simulink model "dcmtrCtrl_PID_Harness2"  (R2022b)
settings: Solver=FixedStepAuto  StartTime=0.0  StopTime=10  FixedStep=Ctrl_Ts  RelTol=1e-3
libraries: simulink_extras x2
settings Model: DataDictionary=dcmtr_ctrl.sldd  Creator=smuckati  LastModifiedBy=smuckati
settings OptimizationCC: DefaultParameterBehavior=Inlined  UseDivisionForNetSlopeComputation=on  EnhancedBackFolding=on  PassReuseOutputArgsAs=Individual arguments  ZeroExternalMemoryAtStartup=off  ZeroInternalMemoryAtStartup=off  OptimizeBlockOrder=speed  DifferentSizesBufferReuse=on  OptimizationCustomize=off  EfficientTunableParamExpr=on
settings DebuggingCC: SignalRangeChecking=error  ParameterPrecisionLossMsg=none  ParameterTunabilityLossMsg=error  UnconnectedInputMsg=warning  UnconnectedOutputMsg=warning  UnconnectedLineMsg=warning
settings ModelReferenceCC: EnableRefExpFcnMdlSchedulingChecks=on
settings SFSimCC: MATLABDynamicMemAlloc=off
settings RTWCC: Description=Embedded Coder  SystemTargetFile=ert.tlc  GenCodeOnly=on  TemplateMakefile=ert_default_tmf  CodeExecutionProfiling=on  CodeProfilingSaveOptions=AllData  CodeProfilingInstrumentation=detailed  DLArmComputeVersion=19.05
settings CodeAppCC: ForceParamTrailComments=on  IgnoreCustomStorageClasses=off  OperatorAnnotations=on  SimulinkDataObjDesc=on  SFDataObjDesc=on  InsertBlockDesc=on
settings ERTTargetCC: TargetLangStandard=C99 (ISO)  GenerateSampleERTMain=on  InlinedParameterPlacement=NonHierarchical  ERTCustomFileTemplate=example_file_process.tlc

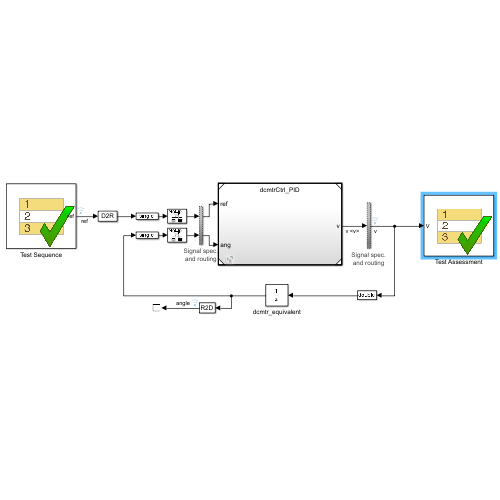
[thumbnail: Simulink's stored preview of the top-level diagram]
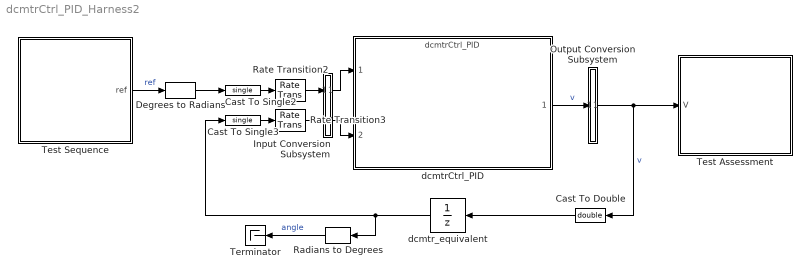
== system dcmtrCtrl_PID_Harness2 ==
  Cast To Double : DataTypeConversion  OutDataTypeStr=double  SaturateOnIntegerOverflow=off  RndMeth=Floor
  Cast To Single2 : DataTypeConversion  OutDataTypeStr=single  SaturateOnIntegerOverflow=off  RndMeth=Floor
  Cast To Single3 : DataTypeConversion  OutDataTypeStr=single  SaturateOnIntegerOverflow=off  RndMeth=Floor
  Degrees to Radians : simulink_extras/Transformations/Degrees to Radians
  Input Conversion Subsystem : Subsystem  Tag=__SLT_ICS__  Description=|
      | Signal spec.
      | and routing
      settings: AttributesFormatString=%<Description>
  Output Conversion Subsystem : Subsystem  Tag=__SLT_OCS__  Description=|
      | Signal spec.
      | and routing
      settings: AttributesFormatString=%<Description>
  Radians to Degrees : simulink_extras/Transformations/Radians to Degrees
  Rate Transition2 : RateTransition  OutPortSampleTime=Ctrl_Ts
  Rate Transition3 : RateTransition  OutPortSampleTime=Ctrl_Ts
  Terminator : Terminator
  Test Assessment : Test Sequence  TreatAsAtomicUnit=on
  Test Sequence : Test Sequence  TreatAsAtomicUnit=on
  dcmtrCtrl_PID : ModelReference  ModelNameDialog=dcmtrCtrl_PID  SimulationMode=Normal  ModelReferenceVersion=3.0
  dcmtr_equivalent : UnitDelay  SampleTime=-1  HasFrameUpgradeWarning=on
  wires:
  Degrees to Radians/1 -> Cast To Single2/1
  Output Conversion Subsystem/1(Outport_1) -> Cast To Double/1, Test Assessment/1(V)  "v"
  Input Conversion Subsystem/1(Outport_1) -> dcmtrCtrl_PID/1
  Input Conversion Subsystem/2(Outport_2) -> dcmtrCtrl_PID/2
  dcmtrCtrl_PID/1 -> Output Conversion Subsystem/1(Inport_1)  "v"
  Cast To Single2/1 -> Rate Transition2/1
  Rate Transition2/1 -> Input Conversion Subsystem/1(Inport_1)
  Cast To Single3/1 -> Rate Transition3/1
  Rate Transition3/1 -> Input Conversion Subsystem/2(Inport_2)
  dcmtr_equivalent/1 -> Radians to Degrees/1, Cast To Single3/1
  Cast To Double/1 -> dcmtr_equivalent/1
  Test Sequence/1(ref) -> Degrees to Radians/1  "ref"
  Radians to Degrees/1 -> Terminator/1  "angle"

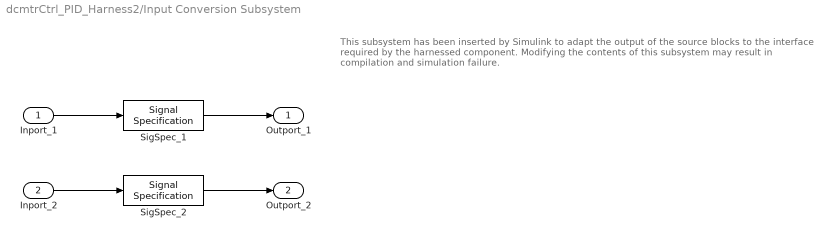
== system dcmtrCtrl_PID_Harness2/Input Conversion Subsystem ==
  note: This subsystem has been inserted by Simulink to adapt the output of the source blocks to the interface required by the harnessed component.
      |  Modifying the contents of this subsystem may result in compilation and simulation failure.
  Inport_1 : Inport
  Inport_2 : Inport  Port=2
  SigSpec_1 : SignalSpecification  OutDataTypeStr=single  Dimensions=[1]  SampleTime=0.01
  SigSpec_2 : SignalSpecification  OutDataTypeStr=single  Dimensions=[1]  SampleTime=0.01
  Outport_1 : Outport
  Outport_2 : Outport  Port=2
  wires:
  SigSpec_1/1 -> Outport_1/1
  Inport_1/1 -> SigSpec_1/1
  SigSpec_2/1 -> Outport_2/1
  Inport_2/1 -> SigSpec_2/1

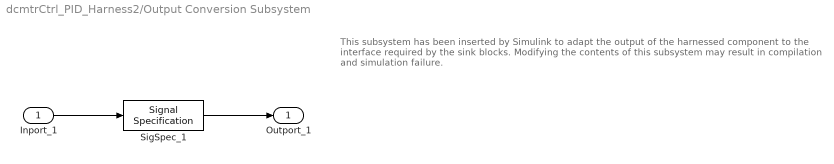
== system dcmtrCtrl_PID_Harness2/Output Conversion Subsystem ==
  note: This subsystem has been inserted by Simulink to adapt the output of the harnessed component to the interface required by the sink blocks.
      |  Modifying the contents of this subsystem may result in compilation and simulation failure.
  Inport_1 : Inport
  SigSpec_1 : SignalSpecification  OutDataTypeStr=single  Dimensions=[1]  SampleTime=0.01
  Outport_1 : Outport
  wires:
  Inport_1/1 -> SigSpec_1/1
  SigSpec_1/1 -> Outport_1/1

== stateflow chart dcmtrCtrl_PID_Harness2/Test Assessment ==
  state MOTOR_REST
  state MONITOR_MAX_VOLT
    verify( abs(V) <= 5)
  (default) -> MOTOR_REST
  MOTOR_REST -> MONITOR_MAX_VOLT : [
      | after(1,sec)
      | ]
  data: V input

== stateflow chart dcmtrCtrl_PID_Harness2/Test Sequence ==
  state MOTOR_INITIALIZE
    ref = pointCalc();
  state INIT_SETUP
    ref = 0;
  state READ_VEHICLEDATA
    ref = pointCalc();
  state FLATTEN
    ref = 0;
  (default) -> MOTOR_INITIALIZE
  MOTOR_INITIALIZE -> INIT_SETUP : [
      | true
      | ]
  INIT_SETUP -> READ_VEHICLEDATA : [
      | after(0.1,sec)
      | ]
  READ_VEHICLEDATA -> FLATTEN : [
      | after(0.5,sec)
      | ]
  FLATTEN -> READ_VEHICLEDATA : [
      | after(0.2,sec)
      | ]
  data: ref output
